simulink model "DLA_Reduced_Bandwidth"  (R2021b)
settings: Solver=VariableStepAuto  StartTime=0.0  StopTime=100  RelTol=1e-3
InitFcn:
  | clc;clear;
  | global Samplesperframe;
  | Samplesperframe = 512;
  | global Upsmp; Upsmp = 8;
  | global D; D = 16;
  | Sampling_time = 1/20e6;
  | RFactor = 0.25;
  | M = 16;
  | global K_DPD; K_DPD = 7;
  | global Q_DPD; Q_DPD = 3;
  | global DPD_coe;
  | DPD_coe = [1;zeros(K_DPD*Q_DPD-1,1)];
  | 
  | global iter; iter = 0;
  | global K_PA; K_PA = 5;
  | global Q_PA; Q_PA = 3;
  | global PA_coe;
  | PA_coe = [1;zeros(K_PA*Q_PA-1,1)];
  | 
  | global flag; flag = 1;
undefined symbols (not defined in the file or in its folder): D, Upsmp
libraries: commfilt2 x1, commrandsrc3 x1, commdigbbndam3 x1
settings Model: Creator=Noether  LastModifiedBy=Noether
settings DataIOCC: ReturnWorkspaceOutputs=off

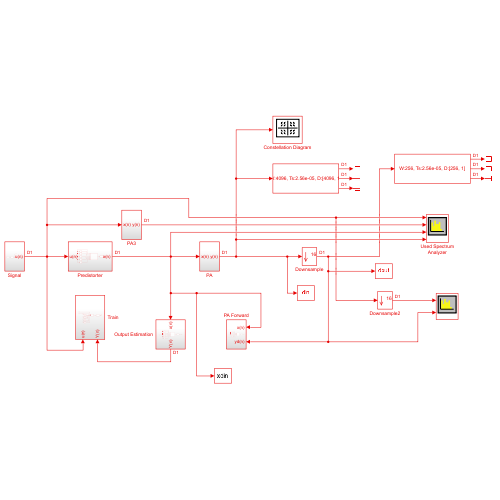
[thumbnail: Simulink's stored preview of the top-level diagram]
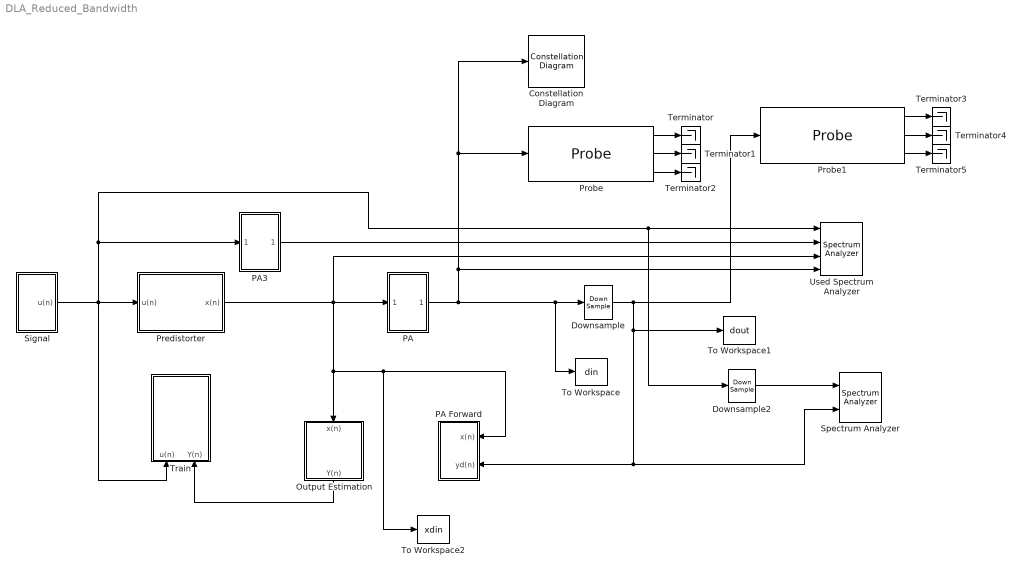
== system DLA_Reduced_Bandwidth ==
  Constellation Diagram : ConstellationDiagram
  Downsample : DownSample  N=D
  Downsample2 : DownSample  N=D
  Output Estimation : Subsystem
  PA : Subsystem
  PA Forward : Subsystem
  PA3 : Subsystem
  Predistorter : Subsystem
  Probe : Probe  ProbeComplexSignal=off  ProbeSignalDimensions=on
  Probe1 : Probe  ProbeComplexSignal=off  ProbeSignalDimensions=on
  Signal : Subsystem
  Spectrum Analyzer : SpectrumAnalyzer  NumInputPorts=2
  Terminator{,1..5} (6 alike) : Terminator
  To Workspace : ToWorkspace  VariableName=din  SampleTime=-1
      settings: MaxDataPoints=4096*D  Save2DSignal=2-D array (concatenate along first dimension)
  To Workspace1 : ToWorkspace  VariableName=dout  SampleTime=-1
      settings: MaxDataPoints=4096  Save2DSignal=2-D array (concatenate along first dimension)
  To Workspace2 : ToWorkspace  VariableName=xdin  SampleTime=-1
      settings: MaxDataPoints=4096*D  Save2DSignal=2-D array (concatenate along first dimension)
  Train : Subsystem
  Used Spectrum Analyzer : SpectrumAnalyzer  NumInputPorts=4
  wires:
  Output Estimation/1(Y(n)) -> Train/2(Y(n))
  Signal/1(u(n)) -> Downsample2/1, Used Spectrum Analyzer/1, PA3/1(x(n)), Train/1(u(n)), Predistorter/1(u(n))
  Predistorter/1(x(n)) -> To Workspace2/1, PA Forward/1(x(n)), Output Estimation/1(x(n)), Used Spectrum Analyzer/3, PA/1(x(n))
  Probe/1 -> Terminator/1
  Probe/2 -> Terminator1/1
  Probe/3 -> Terminator2/1
  Probe1/1 -> Terminator3/1
  PA3/1(y(n)) -> Used Spectrum Analyzer/2
  Probe1/3 -> Terminator5/1
  Probe1/2 -> Terminator4/1
  Downsample/1 -> Spectrum Analyzer/2, PA Forward/2(yd(n)), To Workspace1/1, Probe1/1
  PA/1(y(n)) -> To Workspace/1, Downsample/1, Constellation Diagram/1, Probe/1, Used Spectrum Analyzer/4
  Downsample2/1 -> Spectrum Analyzer/1

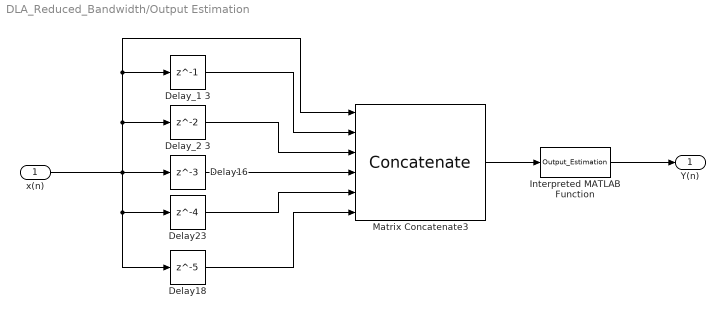
== system DLA_Reduced_Bandwidth/Output Estimation ==
  x(n) : Inport
  Delay16 : Delay  DelayLength=3  InputProcessing=Columns as channels (frame based)
  Delay18 : Delay  DelayLength=5  InputProcessing=Columns as channels (frame based)
  Delay23 : Delay  DelayLength=4  InputProcessing=Columns as channels (frame based)
  Delay_1 3 : Delay  DelayLength=1  InputProcessing=Columns as channels (frame based)
  Delay_2 3 : Delay  InputProcessing=Columns as channels (frame based)
  Interpreted MATLAB Function : MATLABFcn  MATLABFcn=Output_Estimation  Output1D=off
  Matrix Concatenate3 : Concatenate  NumInputs=6  Mode=Multidimensional array  ConcatenateDimension=2
  Y(n) : Outport
  wires:
  Delay_2 3/1 -> Matrix Concatenate3/3
  x(n)/1 -> Delay18/1, Delay23/1, Matrix Concatenate3/1, Delay_1 3/1, Delay_2 3/1, Delay16/1
  Delay18/1 -> Matrix Concatenate3/6
  Delay16/1 -> Matrix Concatenate3/4
  Delay23/1 -> Matrix Concatenate3/5
  Delay_1 3/1 -> Matrix Concatenate3/2
  Matrix Concatenate3/1 -> Interpreted MATLAB Function/1
  Interpreted MATLAB Function/1 -> Y(n)/1

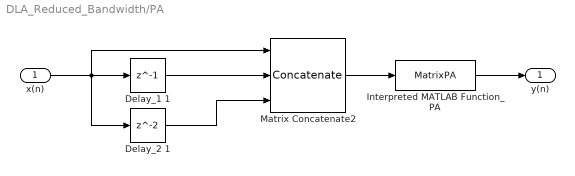
== system DLA_Reduced_Bandwidth/PA ==
  x(n) : Inport
  Delay_1 1 : Delay  DelayLength=1  InputProcessing=Columns as channels (frame based)
  Delay_2 1 : Delay  InputProcessing=Columns as channels (frame based)
  "Interpreted MATLAB Function_PA " : MATLABFcn  MATLABFcn=MatrixPA  Output1D=off
  Matrix Concatenate2 : Concatenate  NumInputs=3  Mode=Multidimensional array  ConcatenateDimension=2
  y(n) : Outport
  wires:
  "Interpreted MATLAB Function_PA "/1 -> y(n)/1
  x(n)/1 -> Delay_2 1/1, Matrix Concatenate2/1, Delay_1 1/1
  Delay_2 1/1 -> Matrix Concatenate2/3
  Matrix Concatenate2/1 -> "Interpreted MATLAB Function_PA "/1
  Delay_1 1/1 -> Matrix Concatenate2/2

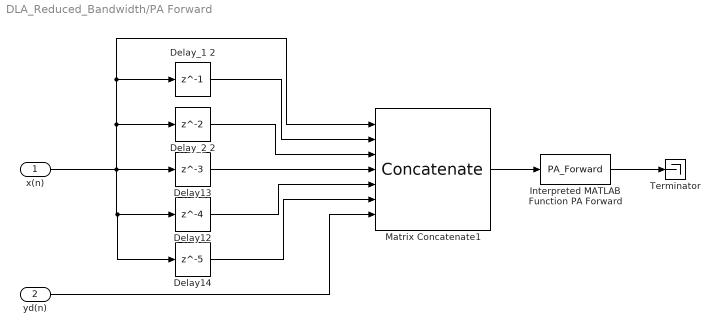
== system DLA_Reduced_Bandwidth/PA Forward ==
  x(n) : Inport
  yd(n) : Inport  Port=2
  Delay12 : Delay  DelayLength=4  InputProcessing=Columns as channels (frame based)
  Delay13 : Delay  DelayLength=3  InputProcessing=Columns as channels (frame based)
  Delay14 : Delay  DelayLength=5  InputProcessing=Columns as channels (frame based)
  Delay_1 2 : Delay  DelayLength=1  InputProcessing=Columns as channels (frame based)
  Delay_2 2 : Delay  InputProcessing=Columns as channels (frame based)
  Interpreted MATLAB Function PA Forward : MATLABFcn  MATLABFcn=PA_Forward  Output1D=off
  Matrix Concatenate1 : Concatenate  NumInputs=7  Mode=Multidimensional array
  Terminator : Terminator
  wires:
  Delay12/1 -> Matrix Concatenate1/5
  x(n)/1 -> Delay13/1, Delay14/1, Delay12/1, Matrix Concatenate1/1, Delay_1 2/1, Delay_2 2/1
  Delay_2 2/1 -> Matrix Concatenate1/3
  Delay14/1 -> Matrix Concatenate1/6
  Delay13/1 -> Matrix Concatenate1/4
  Delay_1 2/1 -> Matrix Concatenate1/2
  Interpreted MATLAB Function PA Forward/1 -> Terminator/1
  Matrix Concatenate1/1 -> Interpreted MATLAB Function PA Forward/1
  yd(n)/1 -> Matrix Concatenate1/7

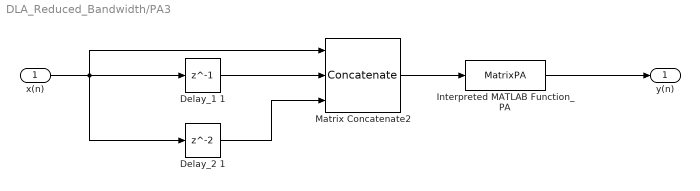
== system DLA_Reduced_Bandwidth/PA3 ==
  x(n) : Inport
  Delay_1 1 : Delay  DelayLength=1  InputProcessing=Columns as channels (frame based)
  Delay_2 1 : Delay  InputProcessing=Columns as channels (frame based)
  "Interpreted MATLAB Function_PA " : MATLABFcn  MATLABFcn=MatrixPA  Output1D=off
  Matrix Concatenate2 : Concatenate  NumInputs=3  Mode=Multidimensional array  ConcatenateDimension=2
  y(n) : Outport
  wires:
  "Interpreted MATLAB Function_PA "/1 -> y(n)/1
  x(n)/1 -> Delay_2 1/1, Matrix Concatenate2/1, Delay_1 1/1
  Delay_2 1/1 -> Matrix Concatenate2/3
  Matrix Concatenate2/1 -> "Interpreted MATLAB Function_PA "/1
  Delay_1 1/1 -> Matrix Concatenate2/2

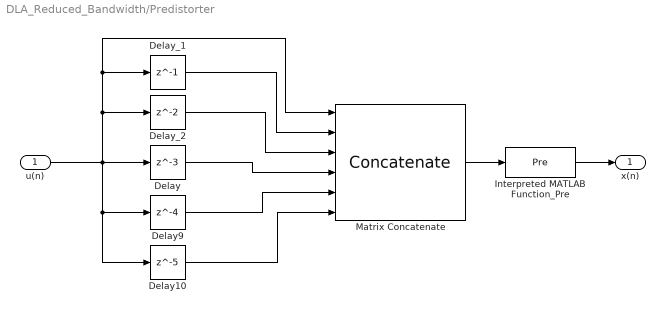
== system DLA_Reduced_Bandwidth/Predistorter ==
  u(n) : Inport
  Delay : Delay  DelayLength=3  InputProcessing=Columns as channels (frame based)
  Delay10 : Delay  DelayLength=5  InputProcessing=Columns as channels (frame based)
  Delay9 : Delay  DelayLength=4  InputProcessing=Columns as channels (frame based)
  "Delay_1 " : Delay  DelayLength=1  InputProcessing=Columns as channels (frame based)
  "Delay_2 " : Delay  InputProcessing=Columns as channels (frame based)
  Interpreted MATLAB Function_Pre : MATLABFcn  MATLABFcn=Pre  Output1D=off
  Matrix Concatenate : Concatenate  NumInputs=6  Mode=Multidimensional array  ConcatenateDimension=2
  x(n) : Outport
  wires:
  Delay/1 -> Matrix Concatenate/4
  u(n)/1 -> Delay9/1, Delay10/1, Delay/1, Matrix Concatenate/1, "Delay_1 "/1, "Delay_2 "/1
  "Delay_1 "/1 -> Matrix Concatenate/2
  Delay9/1 -> Matrix Concatenate/5
  Delay10/1 -> Matrix Concatenate/6
  "Delay_2 "/1 -> Matrix Concatenate/3
  Matrix Concatenate/1 -> Interpreted MATLAB Function_Pre/1
  Interpreted MATLAB Function_Pre/1 -> x(n)/1

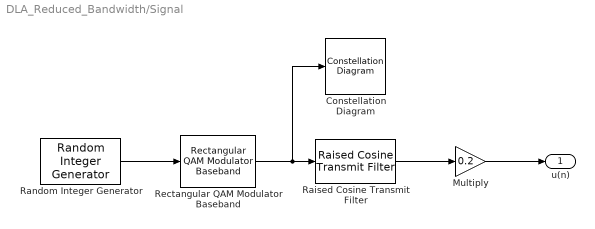
== system DLA_Reduced_Bandwidth/Signal ==
  Constellation Diagram : ConstellationDiagram
  Multiply : Gain  Gain=0.2
  Raised Cosine Transmit Filter : commfilt2/Raised Cosine Transmit Filter  filtType=Square root  R=RFactor  filtSpan=50  N=Upsmp  filterGain=1  InputProcessing=Columns as channels (frame based)  RateOptions=Enforce single-rate processing  framing=Mute  checkCoeff=off  variableName=rcTxFilt  checkGain=Normalized  sampMode=Mute  saveAsFlag=0  currentFiltSpan=50  D=(50)/2  launchFVT=on  roundingMode=Floor  overflowMode=off  coeffDataTypeStr=Inherit: Same word length as input  coeffMin=[]  coeffMax=[]  coeffLastDataTypeStr=Inherit: Same word length as input  outputDataTypeStr=Inherit: Same as accumulator  outputMin=[]  outputMax=[]  outputLastDataTypeStr=Inherit: Same as accumulator
  Random Integer Generator : commrandsrc3/Random Integer Generator  SetSize=M  SeedSource=Parameter  Seed=10  SampleTime=Sampling_time  SamplesPerFrame=Samplesperframe  OutputDataType=double  SimulateUsing=Interpreted execution
  Rectangular QAM Modulator Baseband : commdigbbndam3/Rectangular QAM Modulator Baseband  M=M  InType=Integer  Enc=Gray  Mapping=[0:15]  PowType=Min. distance between symbols  MinDist=2  AvgPow=1  PeakPow=1  Ph=0  outDtype=double  outWordLen=16  outUDDataType=sfix(16)  outFracLenMode=Best precision  outFracLen=15  outDataTypeStr=double  outLastDataTypeStr=double
  u(n) : Outport
  wires:
  Rectangular QAM Modulator Baseband/1 -> Constellation Diagram/1, Raised Cosine Transmit Filter/1
  Random Integer Generator/1 -> Rectangular QAM Modulator Baseband/1
  Raised Cosine Transmit Filter/1 -> Multiply/1
  Multiply/1 -> u(n)/1

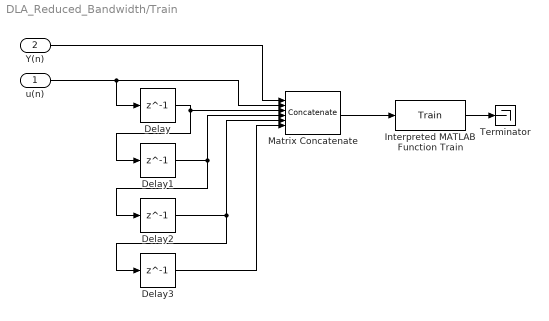
== system DLA_Reduced_Bandwidth/Train ==
  u(n) : Inport
  Y(n) : Inport  Port=2
  Delay{,1..3} (4 alike) : Delay  DelayLength=1  InputProcessing=Columns as channels (frame based)
  Interpreted MATLAB Function Train : MATLABFcn  MATLABFcn=Train
  Matrix Concatenate : Concatenate  NumInputs=6  Mode=Multidimensional array  ConcatenateDimension=2
  Terminator : Terminator
  wires:
  Interpreted MATLAB Function Train/1 -> Terminator/1
  Delay/1 -> Delay1/1, Matrix Concatenate/3
  Y(n)/1 -> Matrix Concatenate/1
  Delay3/1 -> Matrix Concatenate/6
  Matrix Concatenate/1 -> Interpreted MATLAB Function Train/1
  Delay1/1 -> Delay2/1, Matrix Concatenate/4
  u(n)/1 -> Matrix Concatenate/2, Delay/1
  Delay2/1 -> Delay3/1, Matrix Concatenate/5
